simulink model "verify_HeatPump_mdl"  (R2016b)
settings: Solver=ode45  StartTime=0  StopTime=3600  MaxStep=600  RelTol=1e-3  EnableMultiTasking=on
InitFcn:
  | load('DE_TRY2010_13_averageYear')
libraries: carnot x3
settings Model: Creator=drhf  LastModifiedBy=drhf
settings DataIOCC: SaveFormat=Array  SignalLoggingSaveFormat=ModelDataLogs
settings OptimizationCC: ExpressionDepthLimit=2147483647  LifeSpan=inf
settings DebuggingCC: UnderspecifiedInitializationDetection=Classic  MergeDetectMultiDrivingBlocksExec=none  SolverPrmCheckMsg=warning  FcnCallInpInsideContextMsg=warning  StateNameClashWarn=warning  SFUnexpectedBacktrackingDiag=warning  SFNoUnconditionalDefaultTransitionDiag=warning  SFExecutionAtInitializationDiag=none
settings HardwareCC: ProdBitPerPointer=32  ProdBitPerSizeT=32  ProdBitPerPtrDiffT=32  ProdLargestAtomicFloat=None  ProdIntDivRoundTo=Undefined  ProdEndianess=Unspecified  ProdWordSize=32  ProdHWDeviceType=32-bit Generic
settings ModelReferenceCC: PropagateSignalLabelsOutOfModel=off
settings GRTTargetCC: TargetLangStandard=C89/C90 (ANSI)  GeneratePreprocessorConditionals=Disable all  CombineOutputUpdateFcns=off  GRTInterface=on
settings ConfigComp: CovMetricSettings=dw  CovHtmlReporting=on  CovSaveCumulativeToWorkspaceVar=on  CovSaveSingleToWorkspaceVar=on  CovExternalEMLEnable=off

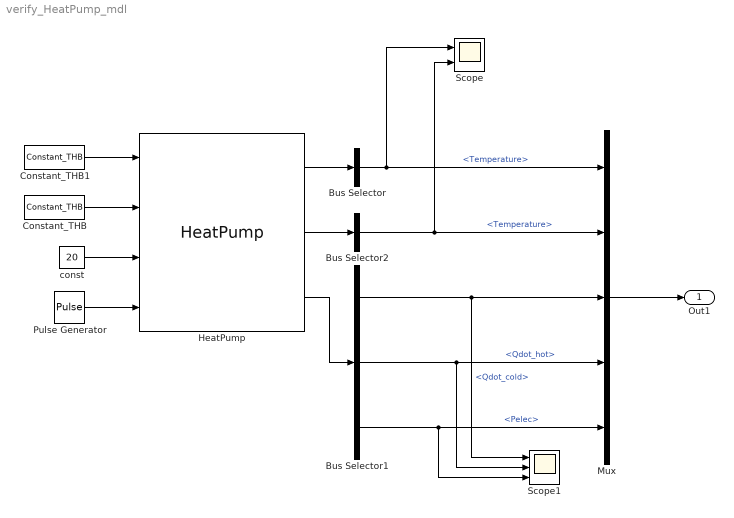
== system verify_HeatPump_mdl ==
  Bus Selector : BusSelector  OutputSignals=Temperature
  Bus Selector1 : BusSelector  OutputSignals=Qdot_cold,Qdot_hot,Pelec
  Bus Selector2 : BusSelector  OutputSignals=Temperature
  Constant_THB : carnot/Source/Simple/Constant_THB  t=40  mdot=2000/3600  p=1e5  mID=No Pressure Drop  fluid=Water  mix=0  mix2=0  mix3=0  dia=0.02  hgt=0
  Constant_THB1 : carnot/Source/Simple/Constant_THB  t=5  mdot=2000/3600  p=1e5  mID=No Pressure Drop  fluid=Water  mix=0  mix2=0  mix3=0  dia=0.02  hgt=0
  HeatPump : carnot/Source/Heat_Pump/HeatPump  Tcin=[-5 15]  Thout=[35 45 55 60]  Qdotc=[14000 12500 10000 9200;26900 24000 21700 20000]  Qdoth=[18000 17200 16500 16000;31500 29500 27800 27000]  Pel=[4400 5500 7000 7500;4600 6000 7000 7500]  caph=80000  capc=50000  UA=7  linc=10  quac=10  linh=10  quah=10
  Mux : Mux  Inputs=5
  Pulse Generator : DiscretePulseGenerator  PulseType=Time based  Period=10*60  PulseWidth=50
  Scope : Scope  NumInputPorts=2
  Scope1 : Scope  NumInputPorts=3
  const : Constant  Value=20
  Out1 : Outport
  wires:
  HeatPump/1 -> Bus Selector/1
  Constant_THB/1 -> HeatPump/2
  Bus Selector/1 -> Mux/1, Scope/1  "<Temperature>"
  HeatPump/2 -> Bus Selector2/1
  const/1 -> HeatPump/3
  Pulse Generator/1 -> HeatPump/4
  Constant_THB1/1 -> HeatPump/1
  HeatPump/3 -> Bus Selector1/1
  Bus Selector2/1 -> Mux/2, Scope/2  "<Temperature>"
  Bus Selector1/3 -> Mux/5, Scope1/3  "<Pelec>"
  Bus Selector1/2 -> Mux/4, Scope1/2  "<Qdot_hot>"
  Bus Selector1/1 -> Mux/3, Scope1/1  "<Qdot_cold>"
  Mux/1 -> Out1/1
